simulink model "size_principle"  (Simulink 7.8)
settings: Solver=ode1  StartTime=0.0  StopTime=10  FixedStep=0.001  RelTol=1e-3
values from neighbouring files (symbols this model uses):
  A = exp(-T/tau)    [emg_filter.m]
  T = 1/1024    (= 0.0009765625)    [emg_filter.m]    (also in get_active_function_coeff.m; set_trfcn.m = 0.001)
  tau = 0.03    [emg_filter.m]
undefined symbols (not defined in the file or in its folder): dfilt, fdesignblkfcn, gcbh, SIZE_MU_1, SIZE_MU_10, SIZE_MU_11, SIZE_MU_12, SIZE_MU_13, SIZE_MU_14, SIZE_MU_15, SIZE_MU_16, SIZE_MU_17, SIZE_MU_18, SIZE_MU_19, SIZE_MU_2, SIZE_MU_20, SIZE_MU_3, SIZE_MU_4, SIZE_MU_5, SIZE_MU_6, SIZE_MU_7, SIZE_MU_8, SIZE_MU_9
libraries: cstblocks x2, simulink x1, dsparch4 x1
settings Model: Creator=minos_niu  LastModifiedBy=minos_niu

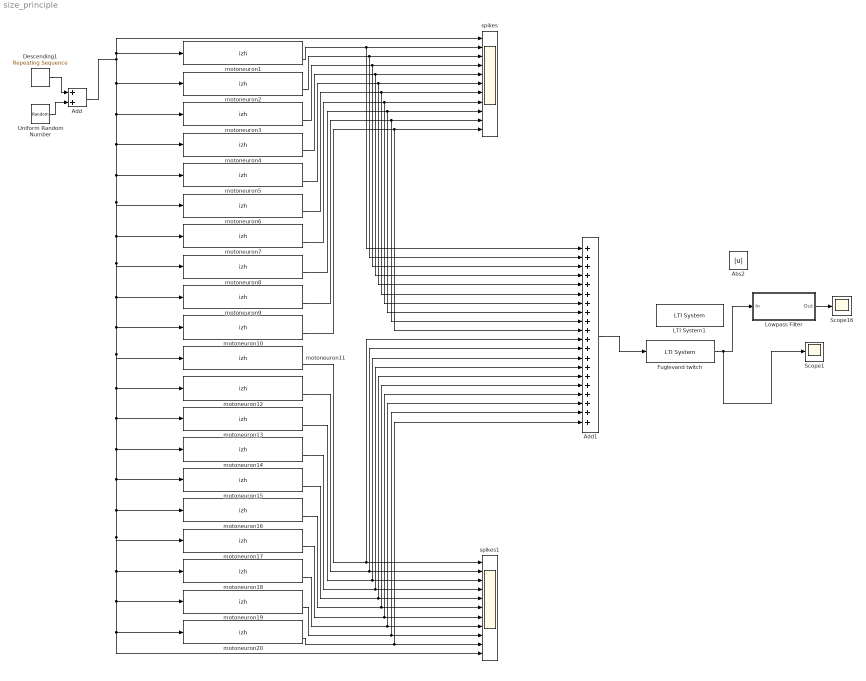
== system size_principle ==
  Abs2 : Abs
  Add : Sum
  Add1 : Sum  Inputs=++++++++++++++++++++
  Descending1 : simulink/Sources/Repeating Sequence  rep_seq_t=[0 1.1 3.1 6.8 9.5 10 ]  rep_seq_y=[0 0 20 20 0 0]*1
  Fuglevand twitch : cstblocks/LTI System  sys=zpk([0], [0.93941 0.93941], 1*2.7183*0.001*0.93941/0.016, 0.001)  IC=[]
  LTI System1 : cstblocks/LTI System  sys=zpk([0], [A A], 2*T*A, T) - zpk([0 -A], [A A A], T^2*A/tau, T)  IC=[]
  Lowpass Filter : Subsystem  DialogController=fdesignblkfcn  DialogControllerArgs=DataTag1  InitFcn=fdesignblkfcn(gcbh, {'InitFcn'});
      settings: CopyFcn=fdesignblkfcn(gcbh, {'CopyFcn'});
      mask Type: Lowpass Filter
      mask Description: Design a lowpass filter
      mask Help: helpview(mapfilelocation('dsp'), 'dsplowpassfilter');
      mask Display: disp('Lowpass')
  Scope1 : Scope
      settings: YMin=0  YMax=450000  SaveName=ScopeData2
  Scope16 : Scope
      settings: TimeRange=10  YMin=0  YMax=350000  SaveName=total_force  DataFormat=Structure
  Uniform Random Number : UniformRandomNumber  Minimum=-6  Maximum=0  SampleTime=0.001
  motoneuron1 : S-Function  FunctionName=izh  Parameters=[0.02 0.2 -65.0 6.0 30.0 SIZE_MU_1] [-70.0 -14.0]  EnableBusSupport=off
      mask Display:
      | port_label('input', 1, 'syn curr');
      | port_label('output', 1, 'action potential');
      | port_label('output', 2, 'spike');
      | disp('Izhi Neuron \n(S-Function)')
  motoneuron10 : S-Function  FunctionName=izh  Parameters=[0.02 0.2 -65.0 6.0 30.0 SIZE_MU_10] [-70.0 -14.0]  EnableBusSupport=off
      mask Display:
      | port_label('input', 1, 'syn curr');
      | port_label('output', 1, 'action potential');
      | port_label('output', 2, 'spike');
      | disp('Izhi Neuron \n(S-Function)')
  motoneuron11 : S-Function  FunctionName=izh  Parameters=[0.02 0.2 -65.0 6.0 30.0 SIZE_MU_11] [-70.0 -14.0]  EnableBusSupport=off
      mask Display:
      | port_label('input', 1, 'syn curr');
      | port_label('output', 1, 'action potential');
      | port_label('output', 2, 'spike');
      | disp('Izhi Neuron \n(S-Function)')
  motoneuron12 : S-Function  FunctionName=izh  Parameters=[0.02 0.2 -65.0 6.0 30.0 SIZE_MU_12] [-70.0 -14.0]  EnableBusSupport=off
      mask Display:
      | port_label('input', 1, 'syn curr');
      | port_label('output', 1, 'action potential');
      | port_label('output', 2, 'spike');
      | disp('Izhi Neuron \n(S-Function)')
  motoneuron13 : S-Function  FunctionName=izh  Parameters=[0.02 0.2 -65.0 6.0 30.0 SIZE_MU_13] [-70.0 -14.0]  EnableBusSupport=off
      mask Display:
      | port_label('input', 1, 'syn curr');
      | port_label('output', 1, 'action potential');
      | port_label('output', 2, 'spike');
      | disp('Izhi Neuron \n(S-Function)')
  motoneuron14 : S-Function  FunctionName=izh  Parameters=[0.02 0.2 -65.0 6.0 30.0 SIZE_MU_14] [-70.0 -14.0]  EnableBusSupport=off
      mask Display:
      | port_label('input', 1, 'syn curr');
      | port_label('output', 1, 'action potential');
      | port_label('output', 2, 'spike');
      | disp('Izhi Neuron \n(S-Function)')
  motoneuron15 : S-Function  FunctionName=izh  Parameters=[0.02 0.2 -65.0 6.0 30.0 SIZE_MU_15] [-70.0 -14.0]  EnableBusSupport=off
      mask Display:
      | port_label('input', 1, 'syn curr');
      | port_label('output', 1, 'action potential');
      | port_label('output', 2, 'spike');
      | disp('Izhi Neuron \n(S-Function)')
  motoneuron16 : S-Function  FunctionName=izh  Parameters=[0.02 0.2 -65.0 6.0 30.0 SIZE_MU_16] [-70.0 -14.0]  EnableBusSupport=off
      mask Display:
      | port_label('input', 1, 'syn curr');
      | port_label('output', 1, 'action potential');
      | port_label('output', 2, 'spike');
      | disp('Izhi Neuron \n(S-Function)')
  motoneuron17 : S-Function  FunctionName=izh  Parameters=[0.02 0.2 -65.0 6.0 30.0 SIZE_MU_17] [-70.0 -14.0]  EnableBusSupport=off
      mask Display:
      | port_label('input', 1, 'syn curr');
      | port_label('output', 1, 'action potential');
      | port_label('output', 2, 'spike');
      | disp('Izhi Neuron \n(S-Function)')
  motoneuron18 : S-Function  FunctionName=izh  Parameters=[0.02 0.2 -65.0 6.0 30.0 SIZE_MU_18] [-70.0 -14.0]  EnableBusSupport=off
      mask Display:
      | port_label('input', 1, 'syn curr');
      | port_label('output', 1, 'action potential');
      | port_label('output', 2, 'spike');
      | disp('Izhi Neuron \n(S-Function)')
  motoneuron19 : S-Function  FunctionName=izh  Parameters=[0.02 0.2 -65.0 6.0 30.0 SIZE_MU_19] [-70.0 -14.0]  EnableBusSupport=off
      mask Display:
      | port_label('input', 1, 'syn curr');
      | port_label('output', 1, 'action potential');
      | port_label('output', 2, 'spike');
      | disp('Izhi Neuron \n(S-Function)')
  motoneuron2 : S-Function  FunctionName=izh  Parameters=[0.02 0.2 -65.0 6.0 30.0 SIZE_MU_2] [-70.0 -14.0]  EnableBusSupport=off
      mask Display:
      | port_label('input', 1, 'syn curr');
      | port_label('output', 1, 'action potential');
      | port_label('output', 2, 'spike');
      | disp('Izhi Neuron \n(S-Function)')
  motoneuron20 : S-Function  FunctionName=izh  Parameters=[0.02 0.2 -65.0 6.0 30.0 SIZE_MU_20] [-70.0 -14.0]  EnableBusSupport=off
      mask Display:
      | port_label('input', 1, 'syn curr');
      | port_label('output', 1, 'action potential');
      | port_label('output', 2, 'spike');
      | disp('Izhi Neuron \n(S-Function)')
  motoneuron3 : S-Function  FunctionName=izh  Parameters=[0.02 0.2 -65.0 6.0 30.0 SIZE_MU_3] [-70.0 -14.0]  EnableBusSupport=off
      mask Display:
      | port_label('input', 1, 'syn curr');
      | port_label('output', 1, 'action potential');
      | port_label('output', 2, 'spike');
      | disp('Izhi Neuron \n(S-Function)')
  motoneuron4 : S-Function  FunctionName=izh  Parameters=[0.02 0.2 -65.0 6.0 30.0 SIZE_MU_4] [-70.0 -14.0]  EnableBusSupport=off
      mask Display:
      | port_label('input', 1, 'syn curr');
      | port_label('output', 1, 'action potential');
      | port_label('output', 2, 'spike');
      | disp('Izhi Neuron \n(S-Function)')
  motoneuron5 : S-Function  FunctionName=izh  Parameters=[0.02 0.2 -65.0 6.0 30.0 SIZE_MU_5] [-70.0 -14.0]  EnableBusSupport=off
      mask Display:
      | port_label('input', 1, 'syn curr');
      | port_label('output', 1, 'action potential');
      | port_label('output', 2, 'spike');
      | disp('Izhi Neuron \n(S-Function)')
  motoneuron6 : S-Function  FunctionName=izh  Parameters=[0.02 0.2 -65.0 6.0 30.0 SIZE_MU_6] [-70.0 -14.0]  EnableBusSupport=off
      mask Display:
      | port_label('input', 1, 'syn curr');
      | port_label('output', 1, 'action potential');
      | port_label('output', 2, 'spike');
      | disp('Izhi Neuron \n(S-Function)')
  motoneuron7 : S-Function  FunctionName=izh  Parameters=[0.02 0.2 -65.0 6.0 30.0 SIZE_MU_7] [-70.0 -14.0]  EnableBusSupport=off
      mask Display:
      | port_label('input', 1, 'syn curr');
      | port_label('output', 1, 'action potential');
      | port_label('output', 2, 'spike');
      | disp('Izhi Neuron \n(S-Function)')
  motoneuron8 : S-Function  FunctionName=izh  Parameters=[0.02 0.2 -65.0 6.0 30.0 SIZE_MU_8] [-70.0 -14.0]  EnableBusSupport=off
      mask Display:
      | port_label('input', 1, 'syn curr');
      | port_label('output', 1, 'action potential');
      | port_label('output', 2, 'spike');
      | disp('Izhi Neuron \n(S-Function)')
  motoneuron9 : S-Function  FunctionName=izh  Parameters=[0.02 0.2 -65.0 6.0 30.0 SIZE_MU_9] [-70.0 -14.0]  EnableBusSupport=off
      mask Display:
      | port_label('input', 1, 'syn curr');
      | port_label('output', 1, 'action potential');
      | port_label('output', 2, 'spike');
      | disp('Izhi Neuron \n(S-Function)')
  spikes : Scope  NumInputPorts=11
      settings: TickLabels=on  TimeRange=5  YMin=-1000~-5~-5~-5~-5~-5~-5~-5~-5~-5~-5  YMax=5000~5~5~5~5~5~5~5~5~5~5  SaveName=spikes_g1  DataFormat=Structure
  spikes1 : Scope  NumInputPorts=11
      settings: TickLabels=on  TimeRange=5  YMin=-1000~-5~-5~-5~-5~-5~-5~-5~-5~-5~-5  YMax=5000~5~5~5~5~5~5~5~5~5~5  SaveName=spikes_g2  DataFormat=Structure
  wires:
  Add/1 -> spikes/1, motoneuron1/1, motoneuron2/1, motoneuron3/1, motoneuron4/1, motoneuron5/1, motoneuron6/1, motoneuron7/1, motoneuron8/1, motoneuron9/1, motoneuron10/1, motoneuron11/1, motoneuron12/1, motoneuron13/1, motoneuron14/1, motoneuron15/1, motoneuron16/1, motoneuron17/1, motoneuron18/1, motoneuron19/1, spikes1/11, motoneuron20/1
  motoneuron1/2 -> spikes/2, Add1/1
  Descending1/1 -> Add/1
  Uniform Random Number/1 -> Add/2
  Lowpass Filter/1(Out) -> Scope16/1
  motoneuron2/2 -> spikes/3, Add1/2
  motoneuron3/2 -> Add1/3, spikes/4
  motoneuron4/2 -> spikes/5, Add1/4
  motoneuron5/2 -> spikes/6, Add1/5
  motoneuron6/2 -> spikes/7, Add1/6
  motoneuron7/2 -> spikes/8, Add1/7
  motoneuron9/2 -> spikes/10, Add1/9
  Fuglevand twitch/1 -> Scope1/1, Lowpass Filter/1(In)
  motoneuron20/2 -> spikes1/10, Add1/20
  motoneuron19/2 -> spikes1/9, Add1/19
  motoneuron18/2 -> spikes1/8, Add1/18
  motoneuron17/2 -> spikes1/7, Add1/17
  motoneuron16/2 -> spikes1/6, Add1/16
  motoneuron15/2 -> spikes1/5, Add1/15
  motoneuron14/2 -> spikes1/4, Add1/14
  motoneuron13/2 -> spikes1/3, Add1/13
  motoneuron12/2 -> spikes1/2, Add1/12
  motoneuron11/2 -> spikes1/1, Add1/11
  motoneuron10/2 -> spikes/11, Add1/10
  Add1/1 -> Fuglevand twitch/1
  motoneuron8/2 -> spikes/9, Add1/8

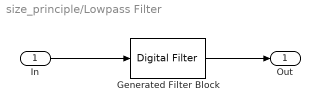
== system size_principle/Lowpass Filter ==
  In : Inport
  Generated Filter Block : dsparch4/Digital Filter  Tag=BlockMethodSubSystem  TypePopup=FIR (all zeros)  IIRFiltStruct=Direct form II transposed  AllPoleFiltStruct=Direct form  FIRFiltStruct=Direct form  CoeffSource=Specify via dialog  NumCoeffs=[0.000595204877442133 0.000254635190406011 0.000308047604271057 0.000367814132296875 0.000434478340747626 0.000508414988635158 0.000590035571175549 0.000679747654269358 0.000777868822071414 0.000884633472779032 0.00100035572983715 0.00112521614601972 0.00125966125920154 0.0014038444034124 0.00155818955783148 0.00172274011508705 0.00189770797205443 0.00208297564909501 0.0022786519245691 0.00248478477740101 0.00270160686757103 0.0029289827639676 0.00316674641779681 0.00341421414193548 0.0036716702932362 0.00393883449431907 0.00421601466996312 0.00450114503951654 0.00479506915687342 0.00509786388878379 0.00540724274319257 0.00572444915888108 0.00604746789391836 0.0063765201295102 0.00671030230122185 0.0070484824019172 0.0073899679144478 0.00773419237306669 0.00808006255844603 0.00842683992849057 0.00877340925258363 0.00911908480028514 0.00946269988278409 0.00980346170608762 0.0101400793790188 0.0104717895372354 0.0107974608415816 0.0111162571259452 0.0114270021557036 0.011728643698953 0.0120203518540101 0.0123012080166268 0.0125702299285631 0.0128265052480324 0.0130690191377833 0.0132974506299961 0.0135103210655435 0.0137075043052072 0.0138879656016236 0.0140512054144866 0.0141967056926303 0.01432377942794 0.0144321325450738 0.0145213248308461 0.014591073590015 0.0146410580526161 0.0146710664886973 0.0146810925552542 0.0146710664886973 0.0146410580526161 0.014591073590015 0.0145213248308461 0.0144321325450738 0.01432377942794 0.0141967056926303 0.0140512054144866 0.0138879656016236 0.0137075043052072 0.0135103210655435 0.0132974506299961 0.0130690191377833 0.0128265052480324 0.0125702299285631 0.0123012080166268 0.0120203518540101 0.011728643698953 0.0114270021557036 0.0111162571259452 0.0107974608415816 0.0104717895372354 0.0101400793790188 0.00980346170608762 0.00946269988278409 0.00911908480028514 0.00877340925258363 0.00842683992849057 0.00808006255844603 0.00773419237306669 0.0073899679144478 0.0070484824019172 0.00671030230122185 0.0063765201295102 0.00604746789391836 0.00572444915888108 0.00540724274319257 0.00509786388878379 0.00479506915687342 0.00450114503951654 0.00421601466996312 0.00393883449431907 0.0036716702932362 0.00341421414193548 0.00316674641779681 0.0029289827639676 0.00270160686757103 0.00248478477740101 0.0022786519245691 0.00208297564909501 0.00189770797205443 0.00172274011508705 0.00155818955783148 0.0014038444034124 0.00125966125920154 0.00112521614601972 0.00100035572983715 0.000884633472779032 0.000777868822071414 0.000679747654269358 0.000590035571175549 0.000508414988635158 0.000434478340747626 0.000367814132296875 0.000308047604271057 0.000254635190406011 0.000595204877442133]  DenCoeffs=[1 0.1]  BiQuadCoeffs=[1 0.3 0.4 1 0.1 0.2]  LatticeCoeffs=[0.2 0.4]  denIgnore=on  FiltPerSampPopup=One filter per frame  IC=0  ICnum=0  ICden=0  roundingMode=Floor  overflowMode=off  ScaleValues=1  scaleValueFracLength=14  stageInFracLength=15  stageOutFracLength=15  FilterSource=Specify via dialog  dfiltObjectName=dfilt.dffir([1 2 1])  InputProcessing=Columns as channels (frame based)
  Out : Outport
  wires:
  Generated Filter Block/1 -> Out/1
  In/1 -> Generated Filter Block/1
